simulink model "linear_beam"  (R2016b)
settings: Solver=VariableStepAuto  StartTime=0.0  StopTime=10.0  RelTol=1e-3
values from neighbouring files (symbols this model uses):
  K_beam = [-8.20687974687 -1.57558991566]    [beam_linearization_controller.mat]    (also in calculate_cascade.m = get(P_beam, 'D'))
libraries: cstblocks x1
settings Model: Creator=piotr  LastModifiedBy=piotr

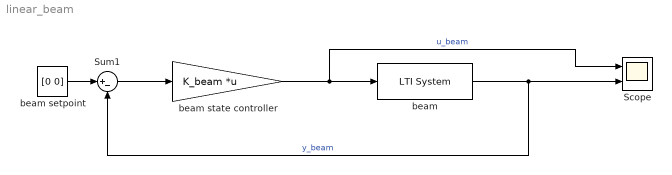
== system linear_beam ==
  Scope : Scope  NumInputPorts=2
  Sum1 : Sum  Inputs=|+-
  beam : cstblocks/LTI System  sys=beam_SS  IC=[-0.3 0]
  beam setpoint : Constant  Value=[0 0]
  beam state controller : Gain  Gain=K_beam  Multiplication=Matrix(K*u) (u vector)
  wires:
  beam state controller/1 -> Scope/1, beam/1  "u_beam"
  beam/1 -> Sum1/2, Scope/2  "y_beam"
  Sum1/1 -> beam state controller/1
  beam setpoint/1 -> Sum1/1
